simulink model "Scenario3"  (R2023a)
settings: Solver=VariableStepAuto  StartTime=0.0  StopTime=30  RelTol=1e-3
libraries: simulink x2
settings Model: Creator=Νίκος  LastModifiedBy=Νίκος

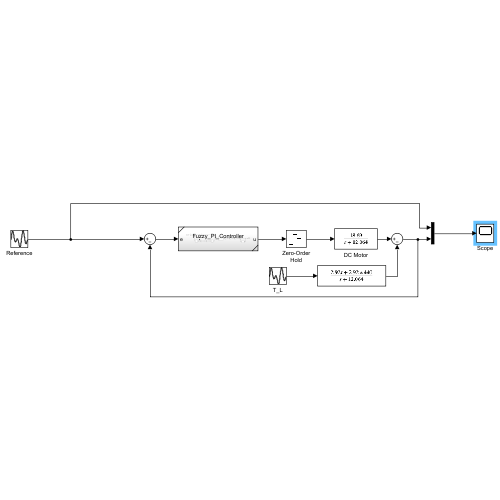
[thumbnail: Simulink's stored preview of the top-level diagram]
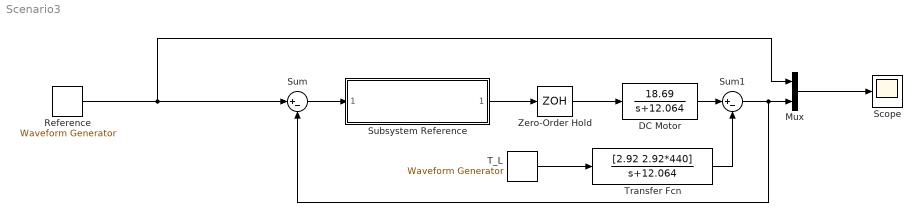
== system Scenario3 ==
  DC Motor : TransferFcn  Numerator=[18.69]  Denominator=[1 12.064]
  Mux : Mux  Inputs=2
  Reference : simulink/Sources/Waveform Generator  OutMin=[]  OutMax=[]  OutDataTypeStr=double  SelectedSignal=1  Signals=step(0,0,150)  BlockNames=MultiportSwitch_91d3b9f81c6f4e7  SampleTime=0.01
  Scope : Scope
  Subsystem Reference : Subsystem  ReferencedSubsystem=Fuzzy_PI_Controller
  Sum : Sum  Inputs=|+-
  Sum1 : Sum  Inputs=|+-
  T_L : simulink/Sources/Waveform Generator  OutMin=[]  OutMax=[]  OutDataTypeStr=double  SelectedSignal=1  Signals=step(10,0,1) - step(20,0,0.5)  BlockNames=MultiportSwitch_8aa6ef4d09d644a  SampleTime=0.01
  Transfer Fcn : TransferFcn  Numerator=[2.92 2.92*440]  Denominator=[1 12.064]
  Zero-Order Hold : ZeroOrderHold  SampleTime=-1
  wires:
  Sum/1 -> Subsystem Reference/1
  Subsystem Reference/1 -> Zero-Order Hold/1
  Sum1/1 -> Mux/2, Sum/2
  Reference/1 -> Mux/1, Sum/1
  Mux/1 -> Scope/1
  Zero-Order Hold/1 -> DC Motor/1
  T_L/1 -> Transfer Fcn/1
  Transfer Fcn/1 -> Sum1/2
  DC Motor/1 -> Sum1/1
